simulink model "simulation_simulink"  (R2019b)
settings: Solver=VariableStepAuto  StartTime=0.0  StopTime=15  RelTol=1e-3
values from neighbouring files (symbols this model uses):
  A = double(round(subs(J_x,   [states, inputs], [trim_state, trim_input])*1000)/1000)    [state_decoupling.m]    (also in state_decouplingv2.m)
  A1_kalman = eval(subs(A1_sampled, t))    [simulation_matlab.m]
  A2_kalman = eval(subs(A2_sampled, t))    [simulation_matlab.m]
  A_s_double = eval(subs(Ad_double,Ts))    [simulation_matlab.m]
  A_s_single = eval(subs(Ad_single,Ts))    [simulation_matlab.m]
  Aaileron = A(6:8,6:8)    [state_decoupling.m]    (also in state_decouplingv2.m = A(5:8,5:8))
  Aelevator = A(2:4,2:4)    [state_decoupling.m]    (also in state_decouplingv2.m = A(1:4,1:4))
  Arudder = A(12,12)    [state_decoupling.m]    (also in state_decouplingv2.m = A(11:12,11:12))
  Athrust = A(9:10,9:10)    [state_decoupling.m]    (also in state_decouplingv2.m)
  B = B*MotorMix    [state_decoupling.m]    (also in state_decouplingv2.m)
  B1_kalman = eval(subs(B1_sampled, t))    [simulation_matlab.m]
  B2_kalman = eval(subs(B2_sampled, t))    [simulation_matlab.m]
  B_s_double = eval(subs(Bd_double,Ts))    [simulation_matlab.m]
  B_s_single = eval(subs(Bd_single,Ts))    [simulation_matlab.m]
  Baileron = B(6:8,3)    [state_decoupling.m]    (also in state_decouplingv2.m = B(5:8,3))
  Belevator = B(2:4,2)    [state_decoupling.m]    (also in state_decouplingv2.m = B(1:4,2))
  Brudder = B(12,4)    [state_decoupling.m]    (also in state_decouplingv2.m = B(11:12,4))
  Bthrust = B(9:10,1)    [state_decoupling.m]    (also in state_decouplingv2.m)
  C = double(round(subs(J_y,   [states, inputs], [trim_state, trim_input])*1000)/1000)    [state_decoupling.m]    (also in state_decouplingv2.m)
  C1_kalman = C1_sampled    [simulation_matlab.m]
  C2_kalman = C2_sampled    [simulation_matlab.m]
  C_double = [1 0]    [simulation_matlab.m]
  C_P = 0.041    [state_decoupling.m]    (also in state_decouplingv2.m)
  C_rollpitch = rho*prop_dia^4*prop_dist/sqrt(2)*[                 1  -1  -1   1 ;                 1   1  -1  -1 ;                 0   0   0   0 ; ]    [state_decoupling.m]    (also in state_decouplingv2.m)
  C_single = [1]    [simulation_matlab.m]
  C_T = [0.069075;4.95e-05]    [state_decoupling.m]    (also in state_decouplingv2.m)
  C_yaw = rho*prop_dia^5/(2*pi)*[                 0   0   0   0 ;                 0   0   0   0 ;                -1   1  -1   1 ; ]    [state_decoupling.m]    (also in state_decouplingv2.m)
  Caileron = [1 0 0; 0 0 1]    [state_decoupling.m]    (also in state_decouplingv2.m = [0 1 0 0; 0 0 0 1])
  Celevator = [1 0 0; 0 0 1]    [state_decoupling.m]    (also in state_decouplingv2.m = [0 1 0 0; 0 0 0 1])
  Crudder = [1]    [state_decoupling.m]    (also in state_decouplingv2.m = [0 1])
  Cthrust = [ 1 0; 0 0]    [state_decoupling.m]    (also in state_decouplingv2.m)
  D = D*MotorMix    [state_decoupling.m]    (also in state_decouplingv2.m)
  D1_kalman = D1_sampled    [simulation_matlab.m]
  D2_kalman = D2_sampled    [simulation_matlab.m]
  D_double = [0]    [simulation_matlab.m]
  D_single = [0]    [simulation_matlab.m]
  Daileron = [0 ; 0]    [state_decoupling.m]    (also in state_decouplingv2.m)
  Delevator = [0 ; 0]    [state_decoupling.m]    (also in state_decouplingv2.m)
  Drudder = 0    [state_decoupling.m]    (also in state_decouplingv2.m)
  Dthrust = [0 ; D(4,1)]    [state_decoupling.m]    (also in state_decouplingv2.m)
  g = [0;0;UAV_mass*9.81]    [state_decoupling.m]    (also in state_decouplingv2.m)
  J = [      Jxx   0   0 ;       0   Jyy  0 ;       0    0  Jzz; ]    [state_decoupling.m]    (also in state_decouplingv2.m)
  Jinv = inv(J)    [state_decoupling.m]    (also in state_decouplingv2.m)
  Kaileron = lqr(Aaileron, Baileron, Qaileron, Raileron)    [simulation_matlab.m]
  Kelevator = lqr(Aelevator, Belevator, Qelevator, Relevator)    [simulation_matlab.m]
  Krudder = lqr(Arudder, Brudder, Qrudder, Rrudder)    [simulation_matlab.m]
  Kthrust = lqr(Athrust, Bthrust, Qthrust, Rthrust)    [simulation_matlab.m]
  M_inv = inv(M_motor)    [simulation_matlab.m]
  M_motor = [1, 1, 1, -1;             1, 1, -1, 1;             1, -1, -1, -1;             1, -1, 1, 1 ]    [simulation_matlab.m]
  measurement_noise = 0.025    [simulation_matlab.m]
  Prop_H = 2*pi*Jprop*[               0  0  0  0 ;               0  0  0  0 ;               1 -1  1 -1 ; ]    [state_decoupling.m]    (also in state_decouplingv2.m)
  q1_noise = 1    [simulation_matlab.m]
  q2_noise = 1    [simulation_matlab.m]
  q3_noise = 1    [simulation_matlab.m]
  q4_noise = 1    [simulation_matlab.m]
  q5_noise = 1    [simulation_matlab.m]
  q_single = cov(out.In_Out_Data{1}.Values.Data)*10000000000000    [simulation_matlab.m]
  r1_noise = 100    [simulation_matlab.m]
  r2_noise = 100    [simulation_matlab.m]
  r3_noise = 100    [simulation_matlab.m]
  r4_noise = 100    [simulation_matlab.m]
  r5_noise = 100    [simulation_matlab.m]
  r_single = cov(out.In_Out_Data{2}.Values.Data)    [simulation_matlab.m]
  tau2 = eval(max(solve(1/sqrt((tau2*2*pi*10)^2+1^2) == 1/sqrt(2), tau2)))    [simulation_matlab.m]
  Thrust_Sum = rho*prop_dia^4*[                 0   0   0   0 ;                 0   0   0   0 ;                -1  -1  -1  -1 ; ]    [state_decoupling.m]    (also in state_decouplingv2.m)
  trim_state = [0,0,0,0,0,0,0,0,0,0,0,0]    [state_decoupling.m]    (also in state_decouplingv2.m)
  Ts = 0.005    [simulation_matlab.m]
  UAV_mass = 0.068    [state_decoupling.m]    (also in state_decouplingv2.m)
undefined symbols (not defined in the file or in its folder): A1_wiener, B1_wiener, C1_wiener, D1_wiener, DiscIntNeverNeededParam, Discrete, L1, Time
libraries: ctrlSharedLib x12, simulink x7, vrlib x3, dspmtrx3 x1
(part 1 of 2)
settings Model: Creator=cwhipp  LastModifiedBy=cwhipp

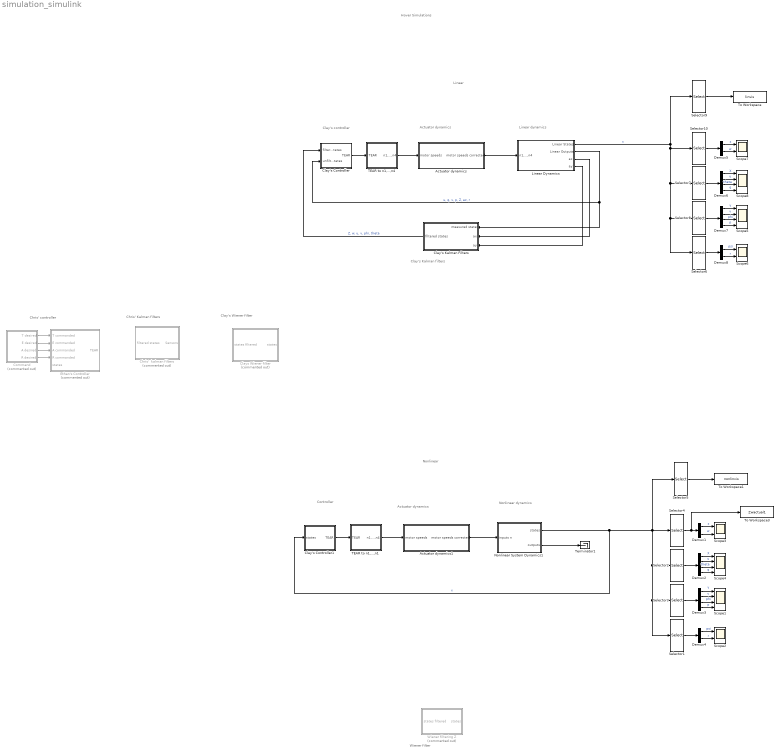
== system simulation_simulink ==
  note: Hover Simulations
  note: Nonlinear
  note: Linear
  note: Clay's controller
  note: Actuator dynamics
  note: Linear dynamics
  note: Clay's Wiener filter
  note: Controller
  note: Actuator dynamics
  note: Nonlinear dynamics
  note: Wiener filter
  note: Chris' Kalman filters
  note: Clay's Kalman filters
  note: Chris' controller
  Actuator dynamics : Subsystem
  Actuator dynamics1 : Subsystem
  Chris'  kalman filters : Subsystem  Commented=on
  Clay's Controller : Subsystem
  Clay's Controller1 : Subsystem
  Clay's Kalman Filters : Subsystem
  Clays Wiener filter : Subsystem  Commented=on
  Command : Subsystem  Commented=on
  Demux{1,4..5,8} (4 alike) : Demux  Outputs=2
  Demux{2..3,6..7} (4 alike) : Demux
  Ethan's Controller : Subsystem  Commented=on
  Linear Dynamics : Subsystem
  Nonlinear System Dynamics1 : Subsystem
  Scope{1,4..5,8} (4 alike) : Scope  NumInputPorts=4
  Scope{2..3,6..7} (4 alike) : Scope  NumInputPorts=2
  Selector1 : Selector  InputPortWidth=12  IndexOptions=Index vector (dialog)  Indices=[11 12]  OutputSizes=1
  Selector10 : Selector  InputPortWidth=12  IndexOptions=Index vector (dialog)  Indices=[1 2]  OutputSizes=1
  Selector2 : Selector  InputPortWidth=12  IndexOptions=Index vector (dialog)  Indices=[3 4 5 6]  OutputSizes=1
  Selector3 : Selector  InputPortWidth=12  IndexOptions=Index vector (dialog)  Indices=[7 8 9 10]  OutputSizes=1
  Selector4 : Selector  InputPortWidth=12  IndexOptions=Index vector (dialog)  Indices=[1 2]  OutputSizes=1
  Selector5 : Selector  InputPortWidth=12  IndexOptions=Index vector (dialog)  Indices=[3 7 1 5 9 11]  OutputSizes=1
  Selector6 : Selector  InputPortWidth=12  IndexOptions=Index vector (dialog)  Indices=[11 12]  OutputSizes=1
  Selector7 : Selector  InputPortWidth=12  IndexOptions=Index vector (dialog)  Indices=[3 4 5 6]  OutputSizes=1
  Selector8 : Selector  InputPortWidth=12  IndexOptions=Index vector (dialog)  Indices=[7 8 9 10]  OutputSizes=1
  Selector9 : Selector  InputPortWidth=12  IndexOptions=Index vector (dialog)  Indices=[3 7 1 5 9 11]  OutputSizes=1
  TEAR to n1,...,n1 : Subsystem
  TEAR to n1,...,n4 : Subsystem
  Terminator1 : Terminator
  To Workspace : ToWorkspace  VariableName=linvis  SampleTime=-1
      settings: Save2DSignal=2-D array (concatenate along first dimension)
  To Workspace1 : ToWorkspace  VariableName=nonlinvis  SampleTime=-1
      settings: Save2DSignal=2-D array (concatenate along first dimension)
  To Workspace3 : ToWorkspace  VariableName=Zwactual1  SaveFormat=Timeseries  SampleTime=-1
  "Wiener filtering Z " : Subsystem  Commented=on
  wires:
  Actuator dynamics1/1(motor speeds corrected) -> Nonlinear System Dynamics1/1(inputs n)
  TEAR to n1,...,n1/1(n1,...,n4) -> Actuator dynamics1/1(motor speeds)
  Nonlinear System Dynamics1/2(outputs) -> Terminator1/1
  Actuator dynamics/1(motor speeds corrected) -> Linear Dynamics/1(n1,...,n4)
  TEAR to n1,...,n4/1(n1,...,n4) -> Actuator dynamics/1(motor speeds)
  Linear Dynamics/2(Linear Outputs) -> Clay's Controller/2(unfiltered states), Clay's Kalman Filters/1(measured states)  "u, q, v, p, Z, az, r"
  Demux4/2 -> Scope2/2  "r"
  Demux3/1 -> Scope1/1  "Y"
  Demux1/1 -> Scope3/1  "z"
  Demux2/4 -> Scope4/4  "q"
  Demux2/3 -> Scope4/3  "theta"
  Demux4/1 -> Scope2/1  "psi"
  Demux2/2 -> Scope4/2  "u"
  Demux1/2 -> Scope3/2  "w"
  Demux3/3 -> Scope1/3  "phi"
  Selector3/1 -> Demux3/1
  Demux2/1 -> Scope4/1  "X"
  Selector1/1 -> Demux4/1
  Selector4/1 -> To Workspace3/1, Demux1/1
  Demux3/4 -> Scope1/4  "p"
  Nonlinear System Dynamics1/1(states) -> Clay's Controller1/1(states), Selector5/1, Selector1/1, Selector3/1, Selector2/1, Selector4/1  "x"
  Selector2/1 -> Demux2/1
  Demux3/2 -> Scope1/2  "v"
  Selector9/1 -> To Workspace/1
  Selector5/1 -> To Workspace1/1
  Command/1(T desired) -> Ethan's Controller/1(T commanded)
  Command/2(E desired) -> Ethan's Controller/2(E commanded)
  Command/3(A desired) -> Ethan's Controller/3(A commanded)
  Command/4(R desired) -> Ethan's Controller/4(R commanded)
  Clay's Controller/1(TEAR) -> TEAR to n1,...,n4/1(TEAR)
  Selector7/1 -> Demux6/1
  Demux7/2 -> Scope5/2  "v"
  Demux6/1 -> Scope8/1  "X"
  Demux6/2 -> Scope8/2  "u"
  Demux7/1 -> Scope5/1  "Y"
  Demux7/3 -> Scope5/3  "phi"
  Demux8/1 -> Scope6/1  "psi"
  Demux5/2 -> Scope7/2  "w"
  Demux7/4 -> Scope5/4  "p"
  Demux8/2 -> Scope6/2  "r"
  Demux6/3 -> Scope8/3  "theta"
  Selector10/1 -> Demux5/1
  Selector8/1 -> Demux7/1
  Demux6/4 -> Scope8/4  "q"
  Selector6/1 -> Demux8/1
  Demux5/1 -> Scope7/1  "z"
  Linear Dynamics/1(Linear States) -> Selector6/1, Selector8/1, Selector7/1, Selector10/1, Selector9/1  "x"
  Clay's Controller1/1(TEAR) -> TEAR to n1,...,n1/1(TEAR)
  Clay's Kalman Filters/1(filtered states) -> Clay's Controller/1(filtered states)  "Z, w, u, v, phi, theta"
  Linear Dynamics/3(ax) -> Clay's Kalman Filters/2(ax)
  Linear Dynamics/4(ay) -> Clay's Kalman Filters/3(ay)

== system simulation_simulink/Actuator dynamics ==
  motor speeds : Inport
  30ms delay : TransportDelay  DelayTime=30e-3
  Demux : Demux
  Mux : Mux
  Saturation4 : Saturate  UpperLimit=500  LowerLimit=10
  Sum : Sum  Inputs=|++
  Sum2 : Sum  Inputs=++|
  Transfer Fcn : TransferFcn  Denominator=[tau2 1]
  Transfer Fcn1 : TransferFcn  Denominator=[tau2 1]
  Transfer Fcn2 : TransferFcn  Denominator=[tau2 1]
  actuator transfer function : TransferFcn  Denominator=[tau2 1]
  process noise : simulink/Sources/Band-Limited White Noise  Commented=on  Cov=0.005*[1; 1; 1; 1]  Ts=0.005  seed=[1; 2; 3; 4]
  speed correction : Constant  Value=293  SampleTime=0.005
  motor speeds corrected : Outport
  wires:
  speed correction/1 -> Sum2/1
  Sum2/1 -> Saturation4/1
  Demux/2 -> Transfer Fcn1/1
  30ms delay/1 -> Demux/1
  Demux/4 -> actuator transfer function/1
  Demux/1 -> Transfer Fcn/1
  Demux/3 -> Transfer Fcn2/1
  Transfer Fcn/1 -> Mux/1
  Transfer Fcn1/1 -> Mux/2
  Transfer Fcn2/1 -> Mux/3
  actuator transfer function/1 -> Mux/4
  Mux/1 -> Sum2/2
  Saturation4/1 -> motor speeds corrected/1
  process noise/1 -> Sum/2
  motor speeds/1 -> Sum/1
  Sum/1 -> 30ms delay/1

== system simulation_simulink/Actuator dynamics1 ==
  motor speeds : Inport
  30ms delay : TransportDelay  DelayTime=30e-3
  Demux : Demux
  Mux : Mux
  Saturation4 : Saturate  UpperLimit=500  LowerLimit=10
  Sum2 : Sum  Inputs=++|
  Transfer Fcn : TransferFcn  Denominator=[tau2 1]
  Transfer Fcn1 : TransferFcn  Denominator=[tau2 1]
  Transfer Fcn2 : TransferFcn  Denominator=[tau2 1]
  actuator transfer function : TransferFcn  Denominator=[tau2 1]
  speed correction : Constant  Value=293
  motor speeds corrected : Outport
  wires:
  speed correction/1 -> Sum2/1
  Sum2/1 -> Saturation4/1
  Demux/2 -> Transfer Fcn1/1
  30ms delay/1 -> Demux/1
  Demux/4 -> actuator transfer function/1
  Demux/1 -> Transfer Fcn/1
  Demux/3 -> Transfer Fcn2/1
  Transfer Fcn/1 -> Mux/1
  Transfer Fcn1/1 -> Mux/2
  Transfer Fcn2/1 -> Mux/3
  actuator transfer function/1 -> Mux/4
  Mux/1 -> Sum2/2
  Saturation4/1 -> motor speeds corrected/1
  motor speeds/1 -> 30ms delay/1

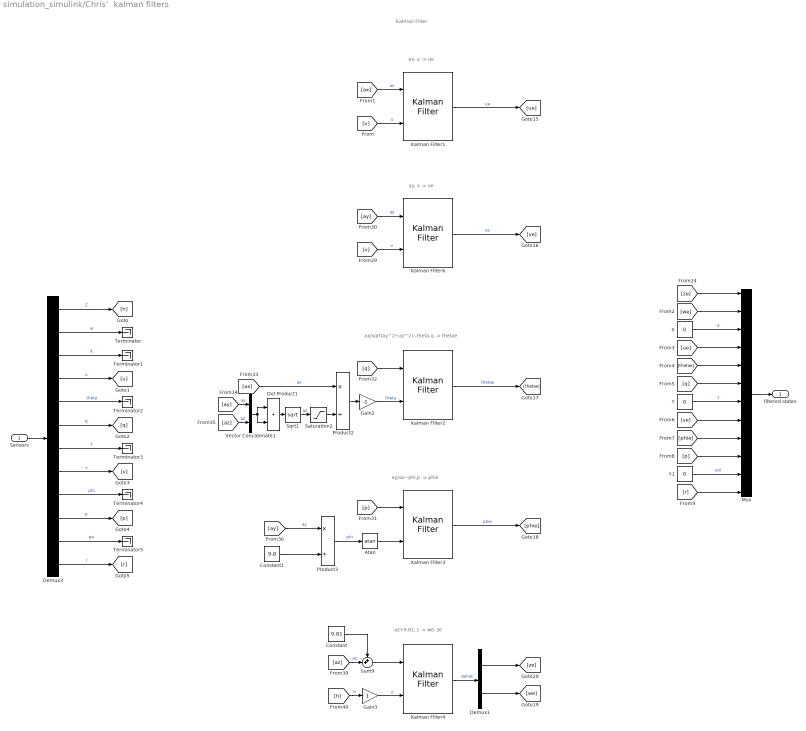
== system simulation_simulink/Chris'  kalman filters ==
  note: Kalman Filter
  note: ay, v -> ve
  note: ax, u -> ue
  note: ax/sqrt(ay^2+az^2)~theta,q -> thetae
  note: ay/az~phi,p -> phie
  note: az+9.81, z -> we, ze
  Sensors : Inport
  Atan : Trigonometry  Operator=atan
  Constant : Constant  Value=9.81
  Constant1 : Constant  Value=9.8
  Demux1 : Demux  Outputs=2
  Demux3 : Demux  Outputs=12
  Dot Product1 : DotProduct  OutMin=0.0001  InputSameDT=on  OutDataTypeStr=Inherit: Inherit via internal rule
  Gain2 : Gain  Gain=-1
  Gain3 : Gain
  Kalman Filter{1..3,6} (4 alike) : ctrlSharedLib/Kalman Filter  TimeDomain=Discrete-Time  UseCurrentEstimator=on  ModelSource=Individual A, B, C, D matrices  ModelSourceVariable=ss(0.95,1,1,0,1)  A=A_s_single  B=B_s_single  C=C_single  D=D_single  NumberOfStates=1  NumberOfInputs=1  NumberOfOutputs=1  InitialEstimateSource=Dialog  X0=[0]  P0=10  UseK=off  UseGH=off  NumberOfProcessNoiseInputs=1  G=1  TimeInvariantG=on  H=0  TimeInvariantH=on  Q=[1]*q_single  TimeInvariantQ=on  R=[1]*r_single*10000  TimeInvariantR=on  N=0  TimeInvariantN=on  AddInputPort=on  AddEnablePort=off  OutputEstimatedY=off  OutputP=off  Ts=Ts
      settings: SourceProductBaseCode=CT
  Kalman Filter4 : ctrlSharedLib/Kalman Filter  TimeDomain=Discrete-Time  UseCurrentEstimator=on  ModelSource=Individual A, B, C, D matrices  ModelSourceVariable=ss(0.95,1,1,0,1)  A=A_s_double  B=B_s_double  C=C_double  D=D_double  NumberOfStates=1  NumberOfInputs=1  NumberOfOutputs=1  InitialEstimateSource=Dialog  X0=[0]  P0=10  UseK=off  UseGH=off  NumberOfProcessNoiseInputs=1  G=1  TimeInvariantG=on  H=0  TimeInvariantH=on  Q=[0 0; 0 1]*q_single  TimeInvariantQ=on  R=[1]*r_single*10000  TimeInvariantR=on  N=0  TimeInvariantN=on  AddInputPort=on  AddEnablePort=off  OutputEstimatedY=off  OutputP=off  Ts=Ts
      settings: SourceProductBaseCode=CT
  Mux : Mux  Inputs=12
  Product2 : Product  Inputs=*/
  Product3 : Product  Inputs=*/
  Saturation2 : Saturate  UpperLimit=inf  LowerLimit=0.001
  Sqrt1 : Sqrt  SaturateOnIntegerOverflow=on
  Sum9 : Sum  Inputs=++|
  Terminator{,1..5} (6 alike) : Terminator
  Vector Concatenate1 : Concatenate
  X : Constant  Value=0  SampleTime=0.005
  Y : Constant  Value=0  SampleTime=0.005
  Y1 : Constant  Value=0  SampleTime=0.005
  filtered states : Outport
  wires:
  [h] -> Gain3/1  "h"
  Kalman Filter1/1 -> [ue]  "ue"
  Kalman Filter6/1 -> [ve]  "ve"
  Kalman Filter2/1 -> [thetae]  "thetae"
  Kalman Filter3/1 -> [phie]  "phie"
  Demux1/2 -> [we]
  Demux1/1 -> [ze]
  Gain3/1 -> Kalman Filter4/2  "z"
  Kalman Filter4/1 -> Demux1/1  "zwhat"
  [ay] -> Product3/1  "ay"
  Product3/1 -> Atan/1  "phi"
  [p] -> Kalman Filter3/1
  [ay] -> Vector Concatenate1/1  "ay"
  [az] -> Vector Concatenate1/2  "az"
  Vector Concatenate1/1 -> Dot Product1/1, Dot Product1/2
  Dot Product1/1 -> Sqrt1/1
  [ax] -> Product2/1  "ax"
  Product2/1 -> Gain2/1
  Sqrt1/1 -> Saturation2/1  "az"
  Saturation2/1 -> Product2/2
  Gain2/1 -> Kalman Filter2/2  "theta"
  [q] -> Kalman Filter2/1
  [ay] -> Kalman Filter6/1  "ay"
  [v] -> Kalman Filter6/2  "v"
  [u] -> Kalman Filter1/2  "u"
  [ax] -> Kalman Filter1/1  "ax"
  [az] -> Sum9/2  "az"
  Sum9/1 -> Kalman Filter4/1
  Constant/1 -> Sum9/1
  Demux3/7 -> Terminator3/1  "Y"
  Demux3/8 -> [v]  "v"
  Demux3/2 -> Terminator/1  "w"
  Demux3/1 -> [h]  "Z"
  Demux3/4 -> [u]  "u"
  Sensors/1 -> Demux3/1
  Demux3/3 -> Terminator1/1  "X"
  Demux3/6 -> [q]  "q"
  Demux3/5 -> Terminator2/1  "theta"
  Demux3/9 -> Terminator4/1  "phi"
  Atan/1 -> Kalman Filter3/2
  Constant1/1 -> Product3/2
  Demux3/10 -> [p]  "p"
  Demux3/11 -> Terminator5/1  "psi"
  Demux3/12 -> [r]  "r"
  [ze] -> Mux/1
  [we] -> Mux/2
  X/1 -> Mux/3  "X"
  [ue] -> Mux/4
  Y/1 -> Mux/7  "Y"
  [ve] -> Mux/8
  [thetae] -> Mux/5
  [q] -> Mux/6
  [phie] -> Mux/9
  [p] -> Mux/10
  Y1/1 -> Mux/11  "psi"
  [r] -> Mux/12
  Mux/1 -> filtered states/1

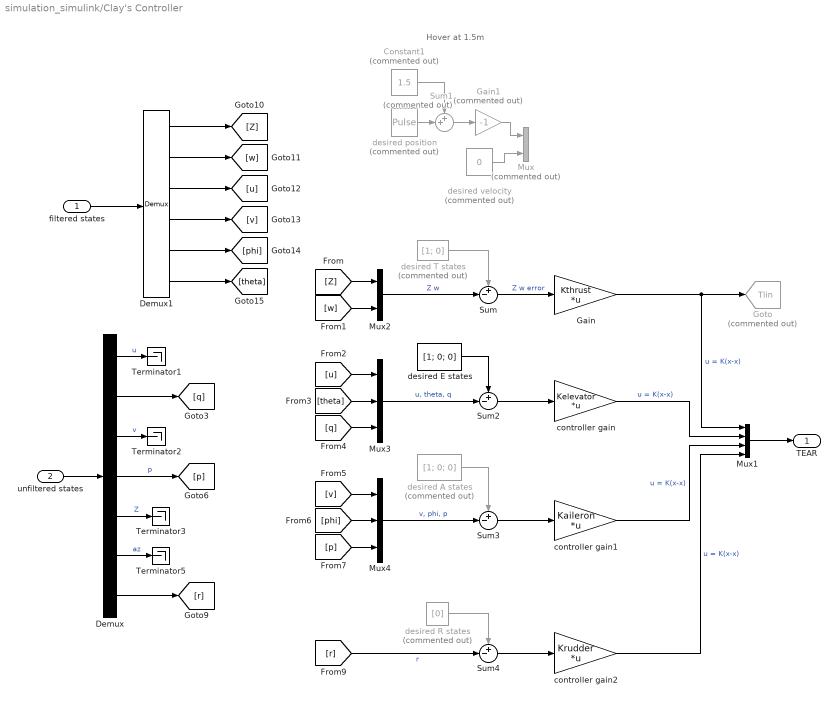
== system simulation_simulink/Clay's Controller ==
  note: Hover at 1.5m
  filtered states : Inport
  unfiltered states : Inport  Port=2
  Constant1 : Constant  Commented=on  Value=1.5  SampleTime=0.05
  Demux : Demux  Outputs=7
  Demux1 : Demux  Outputs=6
  Gain : Gain  Gain=Kthrust  Multiplication=Matrix(K*u)
  Gain1 : Gain  Commented=on  Gain=-1
  Goto : Goto  Commented=on  GotoTag=Tlin  TagVisibility=global
  Mux : Mux  Commented=on  Inputs=2
  Mux1 : Mux
  Mux2 : Mux  Inputs=2
  Mux3 : Mux  Inputs=3
  Mux4 : Mux  Inputs=3
  Sum{,2..4} (4 alike) : Sum  Inputs=+-|
  Sum1 : Sum  Commented=on  Inputs=++|
  Terminator{1..3,5} (4 alike) : Terminator
  controller gain : Gain  Gain=Kelevator  Multiplication=Matrix(K*u)
  controller gain1 : Gain  Gain=Kaileron  Multiplication=Matrix(K*u)
  controller gain2 : Gain  Gain=Krudder  Multiplication=Matrix(K*u)
  desired A states : Constant  Commented=on  Value=[1; 0; 0]  SampleTime=0.005
  desired E states : Constant  Value=[1; 0; 0]  SampleTime=0.005
  desired R states : Constant  Commented=on  Value=[0]  SampleTime=0.005
  desired T states : Constant  Commented=on  Value=[1; 0]  SampleTime=0.005
  desired position : DiscretePulseGenerator  Commented=on  PulseType=Time based  Amplitude=-1.5  Period=10  PulseWidth=50
  desired velocity : Constant  Commented=on  Value=0  SampleTime=0.05
  TEAR : Outport
  wires:
  desired T states/1 -> Sum/1
  Sum/1 -> Gain/1  "Z w error"
  Gain/1 -> Goto/1, Mux1/1  "u = K(x-x)"
  desired E states/1 -> Sum2/1
  Sum2/1 -> controller gain/1
  controller gain/1 -> Mux1/2  "u = K(x-x)"
  controller gain1/1 -> Mux1/3  "u = K(x-x)"
  desired A states/1 -> Sum3/1
  Sum3/1 -> controller gain1/1
  controller gain2/1 -> Mux1/4  "u = K(x-x)"
  Sum4/1 -> controller gain2/1
  desired R states/1 -> Sum4/1
  Mux2/1 -> Sum/2  "Z w"
  Mux3/1 -> Sum2/2  "u, theta, q"
  Mux4/1 -> Sum3/2  "v, phi, p"
  [r] -> Sum4/2  "r"
  Mux1/1 -> TEAR/1
  Sum1/1 -> Gain1/1
  desired position/1 -> Sum1/2
  Gain1/1 -> Mux/1
  desired velocity/1 -> Mux/2
  Constant1/1 -> Sum1/1
  Demux/1 -> Terminator1/1  "u"
  Demux/7 -> [r]
  Demux/6 -> Terminator5/1  "az"
  unfiltered states/1 -> Demux/1
  Demux1/4 -> [v]
  Demux1/6 -> [theta]
  Demux1/3 -> [u]
  Demux1/2 -> [w]
  Demux1/5 -> [phi]
  Demux1/1 -> [Z]
  [Z] -> Mux2/1
  [w] -> Mux2/2
  [u] -> Mux3/1
  [theta] -> Mux3/2
  [q] -> Mux3/3
  [p] -> Mux4/3
  [v] -> Mux4/1
  [phi] -> Mux4/2
  filtered states/1 -> Demux1/1
  Demux/2 -> [q]
  Demux/3 -> Terminator2/1  "v"
  Demux/4 -> [p]  "p"
  Demux/5 -> Terminator3/1  "Z"

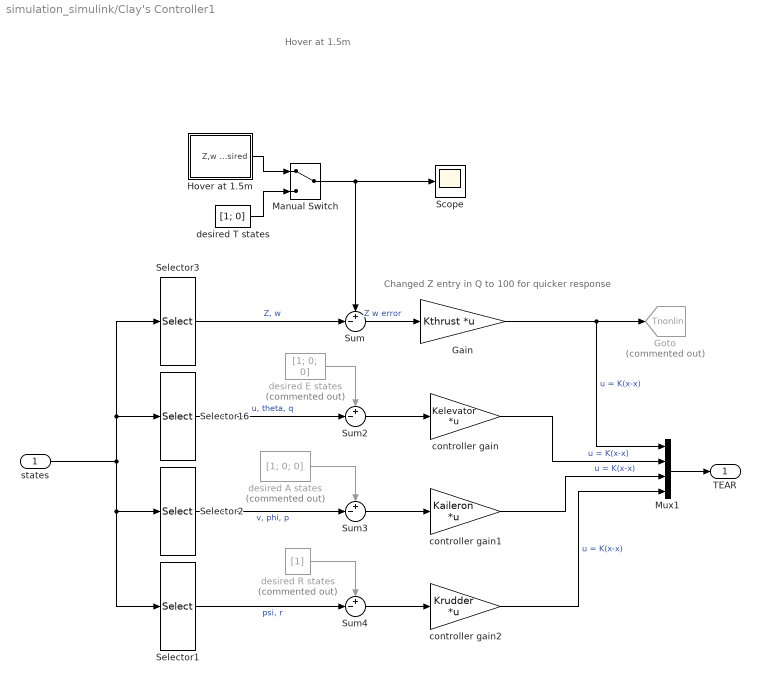
== system simulation_simulink/Clay's Controller1 ==
  note: Changed Z entry in Q to 100 for quicker response
  note: Hover at 1.5m
  states : Inport
  Gain : Gain  Gain=Kthrust  Multiplication=Matrix(K*u)
  Goto : Goto  Commented=on  GotoTag=Tnonlin  TagVisibility=global
  Hover at 1.5m : Subsystem
  Manual Switch : ManualSwitch
  Mux1 : Mux
  Scope : Scope
  Selector1 : Selector  InputPortWidth=12  IndexOptions=Index vector (dialog)  Indices=[12]  OutputSizes=1
  Selector16 : Selector  InputPortWidth=12  IndexOptions=Index vector (dialog)  Indices=[4 5 6]  OutputSizes=1
  Selector2 : Selector  InputPortWidth=12  IndexOptions=Index vector (dialog)  Indices=[8 9 10]  OutputSizes=1
  Selector3 : Selector  InputPortWidth=12  IndexOptions=Index vector (dialog)  Indices=[1 2]  OutputSizes=1
  Sum{,2..4} (4 alike) : Sum  Inputs=+-|
  controller gain : Gain  Gain=Kelevator  Multiplication=Matrix(K*u)
  controller gain1 : Gain  Gain=Kaileron  Multiplication=Matrix(K*u)
  controller gain2 : Gain  Gain=Krudder  Multiplication=Matrix(K*u)
  desired A states : Constant  Commented=on  Value=[1; 0; 0]  VectorParams1D=off  SampleTime=0.005
  desired E states : Constant  Commented=on  Value=[1; 0; 0]  SampleTime=0.005
  desired R states : Constant  Commented=on  Value=[1]  SampleTime=0.005
  desired T states : Constant  Value=[1; 0]  SampleTime=0.005
  TEAR : Outport
  wires:
  states/1 -> Selector16/1, Selector3/1, Selector2/1, Selector1/1
  Sum/1 -> Gain/1  "Z w error"
  Gain/1 -> Goto/1, Mux1/1  "u = K(x-x)"
  desired E states/1 -> Sum2/1
  Sum2/1 -> controller gain/1
  controller gain/1 -> Mux1/2  "u = K(x-x)"
  controller gain1/1 -> Mux1/3  "u = K(x-x)"
  desired A states/1 -> Sum3/1
  Sum3/1 -> controller gain1/1
  controller gain2/1 -> Mux1/4  "u = K(x-x)"
  Sum4/1 -> controller gain2/1
  desired R states/1 -> Sum4/1
  Selector3/1 -> Sum/2  "Z, w"
  Selector16/1 -> Sum2/2  "u, theta, q"
  Selector2/1 -> Sum3/2  "v, phi, p"
  Selector1/1 -> Sum4/2  "psi, r"
  Mux1/1 -> TEAR/1
  Hover at 1.5m/1(Z,w desired) -> Manual Switch/1
  desired T states/1 -> Manual Switch/2
  Manual Switch/1 -> Scope/1, Sum/1

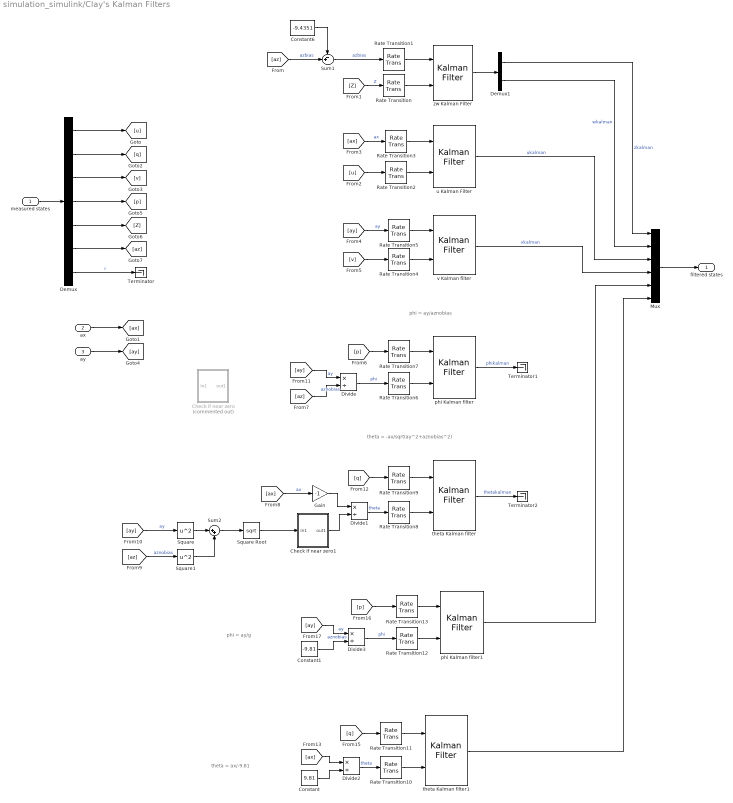
== system simulation_simulink/Clay's Kalman Filters ==
  note: phi = ay/aznobias
  note: theta = -ax/sqrt(ay^2+aznobias^2)
  note: theta = ax/-9.81
  note: phi = ay/g
  measured states : Inport
  ax : Inport  Port=2
  ay : Inport  Port=3
  Check if near zero : Subsystem  Commented=on
  Check if near zero1 : Subsystem
  Constant : Constant  Value=9.81  SampleTime=0.005
  Constant1 : Constant  Value=-9.81  SampleTime=0.005
  Constant6 : Constant  Value=-9.4351
  Demux : Demux  Outputs=7
  Demux1 : Demux  Outputs=2
  Divide{,1..3} (4 alike) : Product  Inputs=*/
  Gain : Gain  Gain=-1
  Mux : Mux  Inputs=6
  Rate Transition{,1..13} (14 alike) : RateTransition  OutPortSampleTime=0.005
  Square : Math  Operator=square  SignedPower=off  SaturateOnIntegerOverflow=on
  Square Root : Sqrt  SaturateOnIntegerOverflow=on
  Square1 : Math  Operator=square  SignedPower=off  SaturateOnIntegerOverflow=on
  Sum1 : Sum  Inputs=-+|
  Sum2 : Sum  Inputs=|++
  Terminator : Terminator
  Terminator1 : Terminator
  Terminator2 : Terminator
  phi Kalman filter : ctrlSharedLib/Kalman Filter  TimeDomain=Discrete-Time  UseCurrentEstimator=on  ModelSource=Individual A, B, C, D matrices  ModelSourceVariable=ss(0.95,1,1,0,1)  A=A2_kalman  B=B2_kalman  C=C2_kalman  D=D2_kalman  NumberOfStates=1  NumberOfInputs=1  NumberOfOutputs=1  InitialEstimateSource=Dialog  X0=[0]  P0=10  UseK=off  UseGH=off  NumberOfProcessNoiseInputs=1  G=1  TimeInvariantG=on  H=0  TimeInvariantH=on  Q=q4_noise;  TimeInvariantQ=on  R=r4_noise;  TimeInvariantR=on  N=0  TimeInvariantN=on  AddInputPort=on  AddEnablePort=off  OutputEstimatedY=off  OutputP=off  Ts=-1
      settings: SourceProductBaseCode=CT
  phi Kalman filter1 : ctrlSharedLib/Kalman Filter  TimeDomain=Discrete-Time  UseCurrentEstimator=on  ModelSource=Individual A, B, C, D matrices  ModelSourceVariable=ss(0.95,1,1,0,1)  A=A2_kalman  B=B2_kalman  C=C2_kalman  D=D2_kalman  NumberOfStates=1  NumberOfInputs=1  NumberOfOutputs=1  InitialEstimateSource=Dialog  X0=[0]  P0=10  UseK=off  UseGH=off  NumberOfProcessNoiseInputs=1  G=1  TimeInvariantG=on  H=0  TimeInvariantH=on  Q=q4_noise;  TimeInvariantQ=on  R=r4_noise;  TimeInvariantR=on  N=0  TimeInvariantN=on  AddInputPort=on  AddEnablePort=off  OutputEstimatedY=off  OutputP=off  Ts=-1
      settings: SourceProductBaseCode=CT
  theta Kalman filter : ctrlSharedLib/Kalman Filter  TimeDomain=Discrete-Time  UseCurrentEstimator=on  ModelSource=Individual A, B, C, D matrices  ModelSourceVariable=ss(0.95,1,1,0,1)  A=A2_kalman  B=B2_kalman  C=C2_kalman  D=D2_kalman  NumberOfStates=1  NumberOfInputs=1  NumberOfOutputs=1  InitialEstimateSource=Dialog  X0=[0]  P0=10  UseK=off  UseGH=off  NumberOfProcessNoiseInputs=1  G=1  TimeInvariantG=on  H=0  TimeInvariantH=on  Q=q5_noise;  TimeInvariantQ=on  R=r5_noise;  TimeInvariantR=on  N=0  TimeInvariantN=on  AddInputPort=on  AddEnablePort=off  OutputEstimatedY=off  OutputP=off  Ts=-1
      settings: SourceProductBaseCode=CT
  theta Kalman filter1 : ctrlSharedLib/Kalman Filter  TimeDomain=Discrete-Time  UseCurrentEstimator=on  ModelSource=Individual A, B, C, D matrices  ModelSourceVariable=ss(0.95,1,1,0,1)  A=A2_kalman  B=B2_kalman  C=C2_kalman  D=D2_kalman  NumberOfStates=1  NumberOfInputs=1  NumberOfOutputs=1  InitialEstimateSource=Dialog  X0=[0]  P0=10  UseK=off  UseGH=off  NumberOfProcessNoiseInputs=1  G=1  TimeInvariantG=on  H=0  TimeInvariantH=on  Q=q5_noise;  TimeInvariantQ=on  R=r5_noise;  TimeInvariantR=on  N=0  TimeInvariantN=on  AddInputPort=on  AddEnablePort=off  OutputEstimatedY=off  OutputP=off  Ts=-1
      settings: SourceProductBaseCode=CT
  u Kalman Filter : ctrlSharedLib/Kalman Filter  TimeDomain=Discrete-Time  UseCurrentEstimator=on  ModelSource=Individual A, B, C, D matrices  ModelSourceVariable=ss(0.95,1,1,0,1)  A=A2_kalman  B=B2_kalman  C=C2_kalman  D=D2_kalman  NumberOfStates=1  NumberOfInputs=1  NumberOfOutputs=1  InitialEstimateSource=Dialog  X0=[0]  P0=10  UseK=off  UseGH=off  NumberOfProcessNoiseInputs=1  G=1  TimeInvariantG=on  H=0  TimeInvariantH=on  Q=q2_noise;  TimeInvariantQ=on  R=r2_noise;  TimeInvariantR=on  N=0  TimeInvariantN=on  AddInputPort=on  AddEnablePort=off  OutputEstimatedY=off  OutputP=off  Ts=-1
      settings: SourceProductBaseCode=CT
  v Kalman filter : ctrlSharedLib/Kalman Filter  TimeDomain=Discrete-Time  UseCurrentEstimator=on  ModelSource=Individual A, B, C, D matrices  ModelSourceVariable=ss(0.95,1,1,0,1)  A=A2_kalman  B=B2_kalman  C=C2_kalman  D=D2_kalman  NumberOfStates=1  NumberOfInputs=1  NumberOfOutputs=1  InitialEstimateSource=Dialog  X0=[0]  P0=10  UseK=off  UseGH=off  NumberOfProcessNoiseInputs=1  G=1  TimeInvariantG=on  H=0  TimeInvariantH=on  Q=q3_noise;  TimeInvariantQ=on  R=r3_noise;  TimeInvariantR=on  N=0  TimeInvariantN=on  AddInputPort=on  AddEnablePort=off  OutputEstimatedY=off  OutputP=off  Ts=-1
      settings: SourceProductBaseCode=CT
  zw Kalman Filter : ctrlSharedLib/Kalman Filter  TimeDomain=Discrete-Time  UseCurrentEstimator=on  ModelSource=Individual A, B, C, D matrices  ModelSourceVariable=ss(0.95,1,1,0,1)  A=A1_kalman  B=B1_kalman  C=C1_kalman  D=D1_kalman  NumberOfStates=1  NumberOfInputs=1  NumberOfOutputs=1  InitialEstimateSource=Dialog  X0=[0;0 ]  P0=10  UseK=off  UseGH=off  NumberOfProcessNoiseInputs=1  G=1  TimeInvariantG=on  H=0  TimeInvariantH=on  Q=[0 0 ; 0 1].*q1_noise;  TimeInvariantQ=on  R=r1_noise;  TimeInvariantR=on  N=0  TimeInvariantN=on  AddInputPort=on  AddEnablePort=off  OutputEstimatedY=off  OutputP=off  Ts=-1
      settings: SourceProductBaseCode=CT
  filtered states : Outport
  wires:
  zw Kalman Filter/1 -> Demux1/1
  Divide1/1 -> Rate Transition8/1  "theta"
  Rate Transition6/1 -> phi Kalman filter/2
  [p] -> Rate Transition7/1
  Sum1/1 -> Rate Transition1/1  "azbias"
  Square/1 -> Sum2/1
  Rate Transition/1 -> zw Kalman Filter/2
  [v] -> Rate Transition4/1
  Demux1/2 -> Mux/2  "wkalman"
  Rate Transition1/1 -> zw Kalman Filter/1
  Rate Transition3/1 -> u Kalman Filter/1
  [q] -> Rate Transition9/1
  Rate Transition4/1 -> v Kalman filter/2
  Gain/1 -> Divide1/1
  [az] -> Divide/2  "aznobias"
  [ax] -> Rate Transition3/1  "ax"
  Rate Transition7/1 -> phi Kalman filter/1
  Rate Transition5/1 -> v Kalman filter/1
  Divide/1 -> Rate Transition6/1  "phi"
  u Kalman Filter/1 -> Mux/3  "ukalman"
  Sum2/1 -> Square Root/1
  [u] -> Rate Transition2/1
  Rate Transition2/1 -> u Kalman Filter/2
  [Z] -> Rate Transition/1  "Z"
  Rate Transition9/1 -> theta Kalman filter/1
  Check if near zero1/1(out1) -> Divide1/2
  Square1/1 -> Sum2/2
  Demux1/1 -> Mux/1  "zkalman"
  v Kalman filter/1 -> Mux/4  "vkalman"
  [ay] -> Rate Transition5/1  "ay"
  Square Root/1 -> Check if near zero1/1(In1)
  Rate Transition8/1 -> theta Kalman filter/2
  measured states/1 -> Demux/1
  Demux/1 -> [u]
  Demux/7 -> Terminator/1  "r"
  [ax] -> Gain/1  "ax"
  [az] -> Square1/1  "aznobias"
  [ay] -> Square/1  "ay"
  [ay] -> Divide/1  "ay"
  Mux/1 -> filtered states/1
  Demux/2 -> [q]
  Demux/3 -> [v]
  Demux/4 -> [p]
  Demux/5 -> [Z]
  Demux/6 -> [az]
  ax/1 -> [ax]
  ay/1 -> [ay]
  [az] -> Sum1/2  "azbias"
  Constant6/1 -> Sum1/1
  [q] -> Rate Transition11/1
  Divide2/1 -> Rate Transition10/1  "theta"
  Rate Transition10/1 -> theta Kalman filter1/2
  Rate Transition11/1 -> theta Kalman filter1/1
  [ax] -> Divide2/1
  Constant/1 -> Divide2/2
  [ay] -> Divide3/1  "ay"
  Divide3/1 -> Rate Transition12/1  "phi"
  Rate Transition12/1 -> phi Kalman filter1/2
  [p] -> Rate Transition13/1
  Rate Transition13/1 -> phi Kalman filter1/1
  Constant1/1 -> Divide3/2  "aznobias"
  phi Kalman filter1/1 -> Mux/5
  theta Kalman filter1/1 -> Mux/6
  phi Kalman filter/1 -> Terminator1/1  "phikalman"
  theta Kalman filter/1 -> Terminator2/1  "thetakalman"

== system simulation_simulink/Clays Wiener filter ==
  states : Inport
  Gain5 : Gain  Gain=-0.067
  Mux : Mux  Inputs=2
  ZNED : Selector  InputPortWidth=12  IndexOptions=Index vector (dialog)  Indices=[1]  OutputSizes=1
  Zw Wiener filter : Subsystem
  states 3-12 : Selector  InputPortWidth=12  IndexOptions=Index vector (dialog)  Indices=[3 4 5 6 7 8 9 10 11 12]  OutputSizes=1
  "states filtered " : Outport
  wires:
  states/1 -> states 3-12/1, ZNED/1
  ZNED/1 -> Zw Wiener filter/2(z)
  Gain5/1 -> Zw Wiener filter/1(az)  "wdot = a_z"
  [Tlin] -> Gain5/1
  Mux/1 -> "states filtered "/1
  Zw Wiener filter/1(zw_wiener) -> Mux/1  "zw"
  states 3-12/1 -> Mux/2

== system simulation_simulink/Command ==
  note: Hover at 1.5m
  Constant1 : Constant  Commented=on  Value=1.5  SampleTime=0.05
  Gain1 : Gain  Commented=on  Gain=-1
  Mux : Mux  Commented=on  Inputs=2
  Sum1 : Sum  Commented=on  Inputs=++|
  desired A states : Constant  Commented=on  Value=[1; 0; 0; 0]  SampleTime=0.005
  desired E states : Constant  Commented=on  Value=[1; 0; 0; 0]  SampleTime=0.005
  desired R states : Constant  Commented=on  Value=[1; 0]  SampleTime=0.005
  desired T states : Constant  Value=[1; 0]  SampleTime=0.005
  desired Z : DiscretePulseGenerator  Commented=on  PulseType=Time based  Amplitude=-1.5  Period=10  PulseWidth=50
  desired w : Constant  Commented=on  Value=0  SampleTime=0.05
  T desired : Outport
  E desired : Outport  Port=2
  A desired : Outport  Port=3
  R desired : Outport  Port=4
  wires:
  desired E states/1 -> E desired/1
  desired A states/1 -> A desired/1
  desired R states/1 -> R desired/1
  desired Z/1 -> Sum1/2
  Gain1/1 -> Mux/1
  Sum1/1 -> Gain1/1
  Constant1/1 -> Sum1/1
  desired w/1 -> Mux/2
  desired T states/1 -> T desired/1

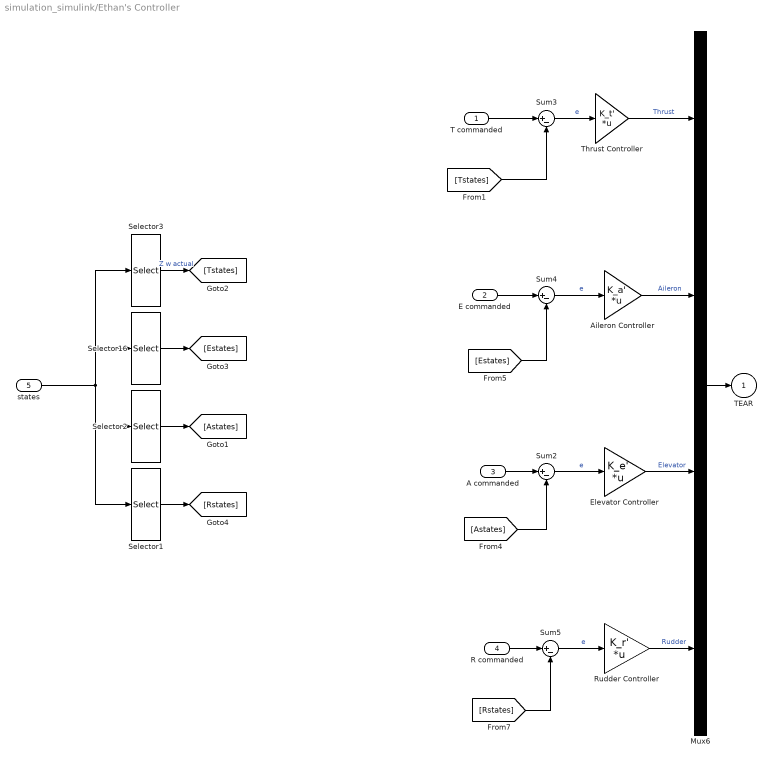
== system simulation_simulink/Ethan's Controller ==
  T commanded : Inport
  E commanded : Inport  Port=2
  A commanded : Inport  Port=3
  R commanded : Inport  Port=4
  states : Inport  Port=5
  Aileron Controller : Gain  Gain=K_a'  Multiplication=Matrix(K*u)
  Elevator Controller : Gain  Gain=K_e'  Multiplication=Matrix(K*u)
  Mux6 : Mux
  Rudder Controller : Gain  Gain=K_r'  Multiplication=Matrix(K*u)
  Selector1 : Selector  InputPortWidth=12  IndexOptions=Index vector (dialog)  Indices=[11 12]  OutputSizes=1
  Selector16 : Selector  InputPortWidth=12  IndexOptions=Index vector (dialog)  Indices=[3 4 5 6]  OutputSizes=1
  Selector2 : Selector  InputPortWidth=12  IndexOptions=Index vector (dialog)  Indices=[7 8 9 10]  OutputSizes=1
  Selector3 : Selector  InputPortWidth=12  IndexOptions=Index vector (dialog)  Indices=[1 2]  OutputSizes=1
  Sum{2..5} (4 alike) : Sum  Inputs=|+-
  Thrust Controller : Gain  Gain=K_t'  Multiplication=Matrix(K*u)
  TEAR : Outport
  wires:
  Mux6/1 -> TEAR/1
  T commanded/1 -> Sum3/1
  [Tstates] -> Sum3/2
  Sum3/1 -> Thrust Controller/1  "e"
  Thrust Controller/1 -> Mux6/1  "Thrust"
  [Astates] -> Sum2/2
  A commanded/1 -> Sum2/1
  E commanded/1 -> Sum4/1
  [Estates] -> Sum4/2
  Sum4/1 -> Aileron Controller/1  "e"
  R commanded/1 -> Sum5/1
  Sum5/1 -> Rudder Controller/1  "e"
  Rudder Controller/1 -> Mux6/4  "Rudder"
  Aileron Controller/1 -> Mux6/2  "Aileron"
  Elevator Controller/1 -> Mux6/3  "Elevator"
  Sum2/1 -> Elevator Controller/1  "e"
  states/1 -> Selector16/1, Selector3/1, Selector2/1, Selector1/1
  Selector3/1 -> [Tstates]  "Z w actual"
  Selector16/1 -> [Estates]
  Selector2/1 -> [Astates]
  Selector1/1 -> [Rstates]
  [Rstates] -> Sum5/2

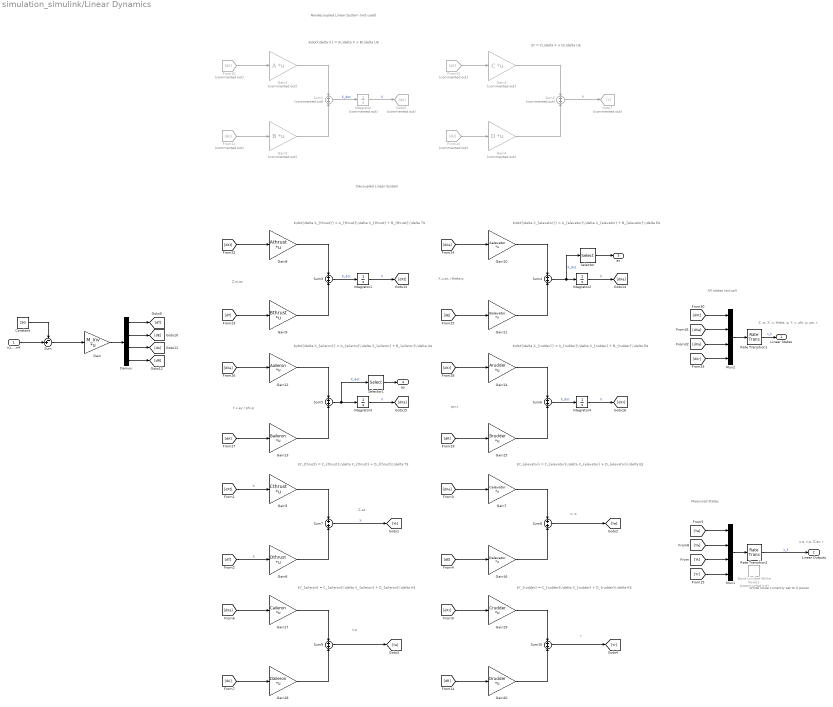
== system simulation_simulink/Linear Dynamics ==
  note: psi,r
  note: Y,v,ay / phi,p
  note: X,u,ax / theta,q
  note: Z,w,az
  note: Decoupled Linear System
  note: $\dot{\delta X} = A\,\delta X + B\,\delta U$
  note: $Y = C\,\delta X + D\,\delta U$
  note: $\dot{\delta X_{thrust}} = A_{thrust}\,\delta X_{thrust} + B_{thrust}\,\delta T$
  note: $\dot{\delta X_{elevator}} = A_{elevator}\,\delta X_{elevator} + B_{elevator}\,\delta E$
  note: $\dot{\delta X_{aileron}} = A_{aileron}\,\delta X_{aileron} + B_{aileron}\,\delta A$
  note: $\dot{\delta X_{rudder}} = A_{rudder}\,\delta X_{rudder} + B_{rudder}\,\delta R$
  note: Z,az
  note: u, q
  note: v,p
  note: r
  note: $Y_{thrust} = C_{thrust}\,\delta X_{thrust} + D_{thrust}\,\delta T$
  note: $Y_{elevator} = C_{elevator}\,\delta X_{elevator} + D_{elevator}\,\delta E$
  note: $Y_{aileron} = C_{aileron}\,\delta X_{aileron} + D_{aileron}\,\delta A$
  note: $Y_{rudder} = C_{rudder}\,\delta X_{rudder} + D_{rudder}\,\delta R$
  note: Nondecoupled Linear System (not used)
  note: All states (actual)
  note: Measured States
  note: u,q, v,p, Z,az, r
  note: Z, w, X, u, theta, q, Y, v, phi, p, psi, r
  note: White noise currently set to 0 power
  n1,...,n4 : Inport
  Band-Limited White Noise1 : simulink/Sources/Band-Limited White Noise  Commented=on  Cov=measurement_noise*ones(9,1)*0  Ts=0.05  seed=[11;12;13;14;15;16;17;18;19]
  Constant : Constant  Value=293
  Demux : Demux
  From10 : From  Commented=on  GotoTag=dX
  From11 : From  Commented=on  GotoTag=dU
  From12 : From  Commented=on  GotoTag=dX
  From13 : From  Commented=on  GotoTag=dU
  Gain : Gain  Gain=M_inv  Multiplication=Matrix(K*u)
  Gain1 : Gain  Commented=on  Gain=A  Multiplication=Matrix(K*u)
  Gain10 : Gain  Gain=Aelevator  Multiplication=Matrix(K*u)
  Gain11 : Gain  Gain=Belevator  Multiplication=Matrix(K*u)
  Gain12 : Gain  Gain=Aaileron  Multiplication=Matrix(K*u)
  Gain13 : Gain  Gain=Baileron  Multiplication=Matrix(K*u)
  Gain14 : Gain  Gain=Arudder  Multiplication=Matrix(K*u)
  Gain15 : Gain  Gain=Brudder  Multiplication=Matrix(K*u)
  Gain16 : Gain  Gain=Delevator  Multiplication=Matrix(K*u)
  Gain17 : Gain  Gain=Caileron  Multiplication=Matrix(K*u)
  Gain18 : Gain  Gain=Daileron  Multiplication=Matrix(K*u)
  Gain19 : Gain  Gain=Crudder  Multiplication=Matrix(K*u)
  Gain2 : Gain  Commented=on  Gain=B  Multiplication=Matrix(K*u)
  Gain20 : Gain  Gain=Drudder  Multiplication=Matrix(K*u)
  Gain3 : Gain  Commented=on  Gain=C  Multiplication=Matrix(K*u)
  Gain4 : Gain  Commented=on  Gain=D  Multiplication=Matrix(K*u)
  Gain5 : Gain  Gain=Cthrust  Multiplication=Matrix(K*u)
  Gain6 : Gain  Gain=Dthrust  Multiplication=Matrix(K*u)
  Gain7 : Gain  Gain=Celevator  Multiplication=Matrix(K*u)
  Gain8 : Gain  Gain=Athrust  Multiplication=Matrix(K*u)
  Gain9 : Gain  Gain=Bthrust  Multiplication=Matrix(K*u)
  Goto5 : Goto  Commented=on  GotoTag=dX
  Goto7 : Goto  Commented=on  GotoTag=Y
  Integrator : Integrator  Commented=on  InitialCondition=trim_state
  Integrator1 : Integrator  InitialCondition=trim_state(9:10)
  Integrator2 : Integrator  InitialCondition=trim_state(1:4)
  Integrator3 : Integrator  InitialCondition=trim_state(5:8)
  Integrator4 : Integrator  InitialCondition=trim_state(11:12)
  Mux1 : Mux
  Mux2 : Mux
  Rate Transition1 : RateTransition  OutPortSampleTime=0.005
  Rate Transition2 : RateTransition  OutPortSampleTime=0.005
  Selector : Selector  InputPortWidth=3  IndexOptions=Index vector (dialog)  Indices=[2]  OutputSizes=1
  Selector1 : Selector  InputPortWidth=3  IndexOptions=Index vector (dialog)  Indices=[2]  OutputSizes=1
  Sum : Sum  Inputs=-+|
  Sum1 : Sum  Commented=on  Inputs=+|+
  Sum{3..10} (8 alike) : Sum  Inputs=+|+
  Sum2 : Sum  Commented=on  Inputs=+|+
  Linear States : Outport
  Linear Outputs : Outport  Port=2
  ax : Outport  Port=3
  ay : Outport  Port=4
  wires:
  Gain14/1 -> Sum6/1
  From11/1 -> Gain2/1
  [dXe] -> Gain10/1
  Gain10/1 -> Sum4/1
  Gain2/1 -> Sum1/2
  Gain15/1 -> Sum6/2
  Gain1/1 -> Sum1/1
  Gain3/1 -> Sum2/1
  Integrator1/1 -> [dXt]  "X"
  From10/1 -> Gain1/1
  Sum1/1 -> Integrator/1  "X_dot"
  Sum2/1 -> Goto7/1  "Y"
  Integrator3/1 -> [dXa]  "X"
  Gain8/1 -> Sum3/1
  [dXt] -> Gain8/1
  Sum3/1 -> Integrator1/1  "X_dot"
  Integrator4/1 -> [dXr]  "X"
  Sum4/1 -> Selector/1, Integrator2/1  "X_dot"
  Gain13/1 -> Sum5/2
  [dXa] -> Gain12/1
  [dXr] -> Gain14/1
  Sum6/1 -> Integrator4/1  "X_dot"
  From13/1 -> Gain4/1
  Gain11/1 -> Sum4/2
  Integrator/1 -> Goto5/1  "X"
  Gain4/1 -> Sum2/2
  Gain12/1 -> Sum5/1
  Integrator2/1 -> [dXe]  "X"
  From12/1 -> Gain3/1
  Gain/1 -> Demux/1
  Demux/3 -> [dA]
  Demux/2 -> [dE]
  Demux/1 -> [dT]
  Demux/4 -> [dR]
  [dXa] -> Mux2/3
  [dXr] -> Mux2/4
  Mux2/1 -> Rate Transition1/1
  [dXt] -> Mux2/1
  [dXe] -> Mux2/2
  Gain6/1 -> Sum7/2
  Gain5/1 -> Sum7/1
  Gain16/1 -> Sum8/2
  [dE] -> Gain16/1
  Gain7/1 -> Sum8/1
  [dXe] -> Gain7/1
  [dA] -> Gain18/1
  Gain17/1 -> Sum9/1
  [dXa] -> Gain17/1
  Gain18/1 -> Sum9/2
  [dXr] -> Gain19/1
  [dR] -> Gain20/1
  Gain20/1 -> Sum10/2
  Gain19/1 -> Sum10/1
  [Ya] -> Mux1/2
  [Ye] -> Mux1/1
  Mux1/1 -> Rate Transition2/1
  [Yr] -> Mux1/4
  [Yt] -> Mux1/3
  [dT] -> Gain9/1
  [dA] -> Gain13/1
  [dR] -> Gain15/1
  [dE] -> Gain11/1
  Sum9/1 -> [Ya]
  Sum10/1 -> [Yr]
  Sum8/1 -> [Ye]
  Gain9/1 -> Sum3/2
  [dT] -> Gain6/1  "X"
  [dXt] -> Gain5/1  "X"
  Sum7/1 -> [Yt]  "X"
  Rate Transition1/1 -> Linear States/1  "x_k"
  Rate Transition2/1 -> Linear Outputs/1  "y_k"
  n1,...,n4/1 -> Sum/2
  Constant/1 -> Sum/1
  Sum/1 -> Gain/1
  Selector/1 -> ax/1
  Sum5/1 -> Selector1/1, Integrator3/1  "X_dot"
  Selector1/1 -> ay/1

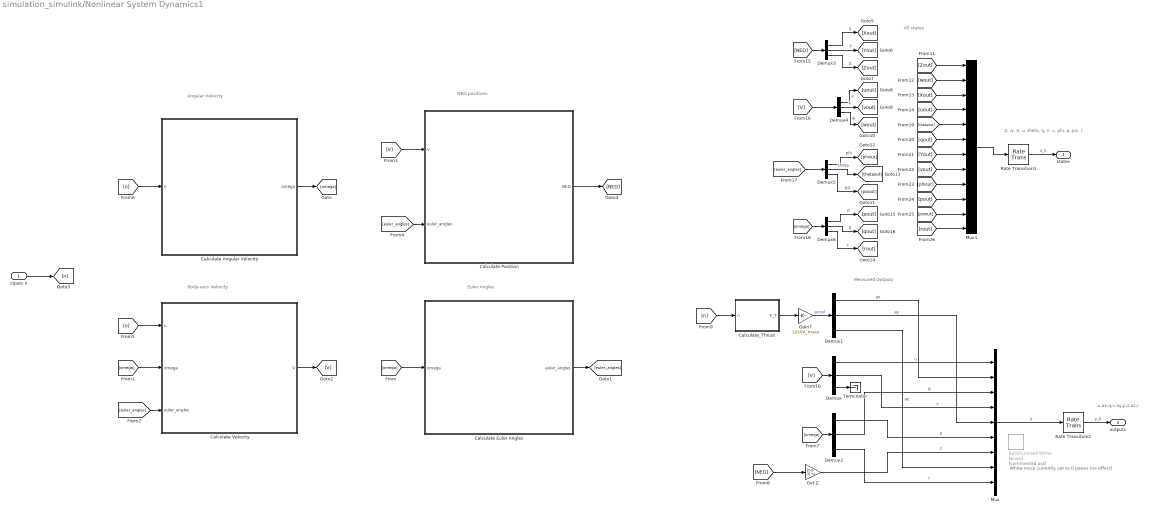
== system simulation_simulink/Nonlinear System Dynamics1 ==
  note: White noise currently set to 0 power (no effect)
  note: Z, w, X, u, theta, q, Y, v, phi, p, psi, r
  note: Euler Angles
  note: NED positions
  note: Angular Velocity
  note: Body-axis Velocity
  note: u,ax,q,v,ay,p,z,az,r
  note: All states
  note: Measured Outputs
  inputs n : Inport
  Band-Limited White Noise1 : simulink/Sources/Band-Limited White Noise  Commented=on  Cov=measurement_noise*ones(9,1)*0  Ts=0.05  seed=[11;12;13;14;15;16;17;18;19]
  Calculate Angular Velocity : Subsystem
  Calculate Euler Angles : Subsystem
  Calculate Position : Subsystem
  Calculate Velocity : Subsystem
  Calculate_Thrust : Subsystem
  Demux{,1..6} (7 alike) : Demux  Outputs=3
  Gain7 : Gain  Gain=1/UAV_mass
      settings: AttributesFormatString=%<Gain>
  Get Z : Gain  Gain=[0 0 -1]  Multiplication=Matrix(K*u)
  Mux : Mux  Inputs=9
  Mux1 : Mux  Inputs=12
  Rate Transition1 : RateTransition  OutPortSampleTime=0.005
  Rate Transition2 : RateTransition  OutPortSampleTime=0.005
  Terminator : Terminator
  states : Outport
  outputs : Outport  Port=2
  wires:
  [euler_angles] -> Demux5/1
  [omega] -> Demux6/1
  Calculate Euler Angles/1(euler_angles) -> [euler_angles]
  [V] -> Calculate Position/1("V ")
  [euler_angles] -> Calculate Position/2(euler_angles)
  Calculate Angular Velocity/1(omega) -> [omega]
  [omega] -> Calculate Euler Angles/1(omega)
  Calculate Velocity/1(V) -> [V]
  [V] -> Demux4/1
  [NED] -> Demux3/1
  [euler_angles] -> Calculate Velocity/3(euler_angles)
  [omega] -> Calculate Velocity/2(omega)
  [n] -> Calculate Velocity/1(n)
  Calculate Position/1(NED) -> [NED]
  [n] -> Calculate Angular Velocity/1(n)
  inputs n/1 -> [n]
  Demux1/1 -> Mux/2  "ax"
  Demux/1 -> Mux/1  "u"
  Mux/1 -> Rate Transition2/1  "y"
  Demux/3 -> Terminator/1
  [omega] -> Demux2/1
  [NED] -> Get Z/1
  Get Z/1 -> Mux/7  "z"
  Demux2/2 -> Mux/3  "q"
  Demux/2 -> Mux/4  "v"
  Demux2/1 -> Mux/6  "p"
  Demux1/2 -> Mux/5  "ay"
  Demux2/3 -> Mux/9  "r"
  [V] -> Demux/1
  Demux1/3 -> Mux/8  "az"
  Gain7/1 -> Demux1/1  "accel"
  Calculate_Thrust/1(F_T) -> Gain7/1
  [n] -> Calculate_Thrust/1(n)
  Rate Transition1/1 -> states/1  "x_k"
  Rate Transition2/1 -> outputs/1  "y_k"
  Mux1/1 -> Rate Transition1/1
  Demux3/1 -> [Xout]  "X"
  Demux3/2 -> [Yout]  "Y"
  Demux3/3 -> [Zout]  "Z"
  Demux4/1 -> [uout]  "u"
  Demux4/2 -> [vout]  "V"
  Demux4/3 -> [wout]  "w"
  Demux5/1 -> [phiout]  "phi"
  Demux5/2 -> [thetaout]  "theta"
  Demux5/3 -> [psiout]  "psi"
  Demux6/1 -> [pout]  "p"
  Demux6/2 -> [qout]  "q"
  Demux6/3 -> [rout]  "r"
  [Zout] -> Mux1/1
  [wout] -> Mux1/2
  [rout] -> Mux1/12
  [psiout] -> Mux1/11
  [pout] -> Mux1/10
  [phiout] -> Mux1/9
  [vout] -> Mux1/8
  [Yout] -> Mux1/7
  [qout] -> Mux1/6
  [uout] -> Mux1/4
  [Xout] -> Mux1/3
  [thetaout] -> Mux1/5

== system simulation_simulink/TEAR to n1,...,n1 ==
  TEAR : Inport
  Convert fom TEAR to n1,..,n4 : Gain  Gain=M_motor  Multiplication=Matrix(K*u)
  n1,...,n4 : Outport
  wires:
  Convert fom TEAR to n1,..,n4/1 -> n1,...,n4/1
  TEAR/1 -> Convert fom TEAR to n1,..,n4/1

== system simulation_simulink/TEAR to n1,...,n4 ==
  TEAR : Inport
  Convert fom TEAR to n1,..,n4 : Gain  Gain=M_motor  Multiplication=Matrix(K*u)
  n1,...,n4 : Outport
  wires:
  Convert fom TEAR to n1,..,n4/1 -> n1,...,n4/1
  TEAR/1 -> Convert fom TEAR to n1,..,n4/1

== system simulation_simulink/Wiener filtering Z  ==
  states : Inport
  Demux : Demux  Outputs=2
  Gain5 : Gain  Gain=-0.067
  Mux : Mux  Inputs=5
  ZNED : Selector  InputPortWidth=12  IndexOptions=Index vector (dialog)  Indices=[3]  OutputSizes=1
  states 1 2 : Selector  InputPortWidth=12  IndexOptions=Index vector (dialog)  Indices=[1 2]  OutputSizes=1
  "states 4, 5" : Selector  InputPortWidth=12  IndexOptions=Index vector (dialog)  Indices=[4 5]  OutputSizes=1
  states 7-12 : Selector  InputPortWidth=12  IndexOptions=Index vector (dialog)  Indices=[7 8 9 10 11 12]  OutputSizes=1
  zw wiener filter2 : Subsystem
  "states filtered " : Outport
  wires:
  "states 4, 5"/1 -> Mux/3
  states 1 2/1 -> Mux/1
  states/1 -> states 7-12/1, "states 4, 5"/1, ZNED/1, states 1 2/1
  ZNED/1 -> zw wiener filter2/2(z)
  Gain5/1 -> zw wiener filter2/1(az)  "wdot = a_z"
  [Tnonlin] -> Gain5/1
  Mux/1 -> "states filtered "/1
  zw wiener filter2/1(zw_wiener) -> Demux/1  "zw"
  Demux/1 -> Mux/2
  Demux/2 -> Mux/4
  states 7-12/1 -> Mux/5

== system simulation_simulink/Clay's Controller1/Hover at 1.5m ==
  Constant1 : Constant  Value=1.5  SampleTime=0.05
  Gain1 : Gain  Gain=-1
  Mux : Mux  Inputs=2
  Sum1 : Sum  Inputs=++|
  desired position : DiscretePulseGenerator  PulseType=Time based  Amplitude=-1.5  Period=10  PulseWidth=50
  desired velocity : Constant  Value=0  SampleTime=0.05
  Z,w desired : Outport
  wires:
  Gain1/1 -> Mux/1
  desired position/1 -> Sum1/2
  Constant1/1 -> Sum1/1
  Sum1/1 -> Gain1/1
  desired velocity/1 -> Mux/2
  Mux/1 -> Z,w desired/1

== system simulation_simulink/Clay's Kalman Filters/Check if near zero ==
  In1 : Inport
  Check sign of input : Switch  Criteria=u2 > Threshold
  Constant3 : Constant  Value=0.5  SampleTime=0.005
  Constant4 : Constant  Value=-0.5  SampleTime=0.005
  Decide what to input : Switch  Criteria=u2 > Threshold
  Interval Test : simulink/Logic and Bit Operations/Interval Test  IntervalClosedRight=on  uplimit=0.5  IntervalClosedLeft=on  lowlimit=-0.5  OutDataTypeStr=boolean
  To Workspace1 : ToWorkspace  VariableName=checksign  SaveFormat=Structure With Time  SampleTime=-1
  To Workspace2 : ToWorkspace  VariableName=booleanoutput1  SaveFormat=Structure With Time  SampleTime=-1
  To Workspace8 : ToWorkspace  VariableName=booleanoutput  SaveFormat=Structure With Time  SampleTime=-1
  out1 : Outport
  wires:
  Decide what to input/1 -> To Workspace2/1, out1/1  "a_z"
  Interval Test/1 -> To Workspace8/1, Decide what to input/2
  Check sign of input/1 -> Decide what to input/1, To Workspace1/1
  In1/1 -> Check sign of input/2, Interval Test/1, Decide what to input/3
  Constant4/1 -> Check sign of input/3
  Constant3/1 -> Check sign of input/1

== system simulation_simulink/Clay's Kalman Filters/Check if near zero1 ==
  In1 : Inport
  Check sign of input : Switch  Criteria=u2 > Threshold
  Constant3 : Constant  Value=0.5  SampleTime=0.005
  Constant4 : Constant  Value=-0.5  SampleTime=0.005
  Decide what to input : Switch  Criteria=u2 > Threshold
  Interval Test : simulink/Logic and Bit Operations/Interval Test  IntervalClosedRight=on  uplimit=0.5  IntervalClosedLeft=on  lowlimit=-0.5  OutDataTypeStr=boolean
  To Workspace : ToWorkspace  VariableName=possiblezero2  SaveFormat=Structure With Time  SampleTime=-1
  out1 : Outport
  wires:
  Decide what to input/1 -> To Workspace/1, out1/1  "a_z"
  Interval Test/1 -> Decide what to input/2
  Check sign of input/1 -> Decide what to input/1
  In1/1 -> Check sign of input/2, Interval Test/1, Decide what to input/3
  Constant4/1 -> Check sign of input/3
  Constant3/1 -> Check sign of input/1

== system simulation_simulink/Clays Wiener filter/Zw Wiener filter ==
  note: zw Wiener Filter
  az : Inport
  z : Inport  Port=2
  Discrete-Time Integrator : DiscreteIntegrator  SampleTime=-1  ICPrevOutput=DiscIntNeverNeededParam  ICPrevScaledInput=DiscIntNeverNeededParam
  Gain1 : Gain  Gain=A1_wiener  Multiplication=Matrix(K*u)
  Gain2 : Gain  Gain=B1_wiener  Multiplication=Matrix(K*u)
  Gain3 : Gain  Gain=L1  Multiplication=Matrix(K*u)
  Gain4 : Gain  Gain=C1_wiener  Multiplication=Matrix(K*u)
  Gain6 : Gain  Gain=D1_wiener  Multiplication=Matrix(K*u)
  Sum : Sum  Inputs=|++
  Sum3 : Sum  Inputs=+++
  Sum7 : Sum  Inputs=-+-
  process noise : simulink/Sources/Band-Limited White Noise  Commented=on  Cov=0.005  Ts=0.005  seed=[1]
  zw_wiener : Outport
  wires:
  Gain3/1 -> Sum3/3  "L(y-Cx-Du)"
  Gain1/1 -> Sum3/1  "Axe"
  Gain2/1 -> Sum3/2  "Bu"
  Discrete-Time Integrator/1 -> zw_wiener/1, Gain1/1, Gain4/1  "xe"
  Gain6/1 -> Sum7/1  "Du"
  Sum7/1 -> Gain3/1
  z/1 -> Sum7/2  "Zned"
  Gain4/1 -> Sum7/3  "Cx"
  Sum3/1 -> Discrete-Time Integrator/1
  process noise/1 -> Sum/2
  az/1 -> Sum/1  "u = az"
  Sum/1 -> Gain6/1, Gain2/1

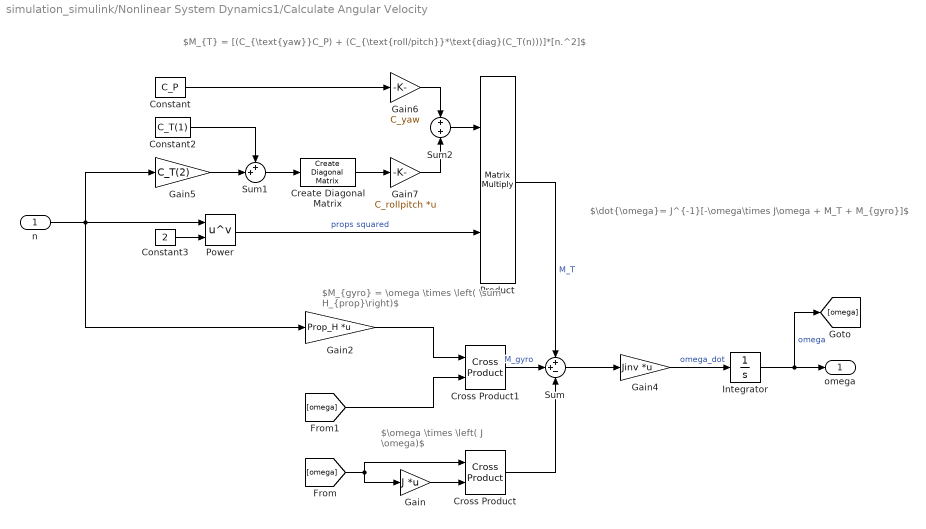
== system simulation_simulink/Nonlinear System Dynamics1/Calculate Angular Velocity ==
  note: $M_{gyro} = \omega \times \left( \sum H_{prop}\right)$
  note: $\dot{\omega}= J^{-1}[-\omega\times J\omega + M_T + M_{gyro}]$
  note: $\omega \times \left( J \omega)$
  note: $M_{T} = [(C_{\text{yaw}}C_P) + (C_{\text{roll/pitch}}*\text{diag}(C_T(n)))]*[n.^2]$
  n : Inport
  Constant : Constant  Value=C_P
  Constant2 : Constant  Value=C_T(1)
  Constant3 : Constant  Value=2
  Create Diagonal Matrix : dspmtrx3/Create Diagonal Matrix
      settings: SourceProductName=DSP System Toolbox  SourceProductBaseCode=DS
  Cross Product : vrlib/Utilities/Cross Product
      settings: SourceProductName=Simulink
  Cross Product1 : vrlib/Utilities/Cross Product
      settings: SourceProductName=Simulink
  Gain : Gain  Gain=J  Multiplication=Matrix(K*u)
  Gain2 : Gain  Gain=Prop_H  Multiplication=Matrix(K*u)
  Gain4 : Gain  Gain=Jinv  Multiplication=Matrix(K*u)
      settings: AttributesFormatString=%<Gain>
  Gain5 : Gain  Gain=C_T(2)
  Gain6 : Gain  Gain=C_yaw
      settings: AttributesFormatString=%<Gain>
  Gain7 : Gain  Gain=C_rollpitch  Multiplication=Matrix(K*u)
      settings: AttributesFormatString=%<Gain>
  Integrator : Integrator  InitialCondition=[0;0;0]
  Power : Math  Operator=pow  SignedPower=off  SaturateOnIntegerOverflow=on
  Product : Product  Multiplication=Matrix(*)
  Sum : Sum  Inputs=++-
  Sum1 : Sum  Inputs=++|
  Sum2 : Sum  Inputs=+|+
  omega : Outport
  wires:
  Sum/1 -> Gain4/1
  [omega] -> Gain/1, Cross Product/1
  Cross Product/1 -> Sum/3
  [omega] -> Cross Product1/2
  Gain2/1 -> Cross Product1/1
  Cross Product1/1 -> Sum/2  "M_gyro"
  Gain4/1 -> Integrator/1  "omega_dot"
  Gain/1 -> Cross Product/2
  Integrator/1 -> [omega], omega/1  "omega"
  Product/1 -> Sum/1  "M_T"
  Create Diagonal Matrix/1 -> Gain7/1
  Sum2/1 -> Product/1
  Sum1/1 -> Create Diagonal Matrix/1
  Constant/1 -> Gain6/1
  Power/1 -> Product/2  "props squared"
  Gain6/1 -> Sum2/1
  Gain5/1 -> Sum1/2
  Gain7/1 -> Sum2/2
  n/1 -> Gain2/1, Power/1, Gain5/1
  Constant2/1 -> Sum1/1
  Constant3/1 -> Power/2
